simulink model "model"  (R2023b)
settings: Solver=ode23s  StartTime=0.0  StopTime=Tsim  MaxStep=1  RelTol=1e-3
values from neighbouring files (symbols this model uses):
  battery_capacity = 58    [parameters.m]    (also in vehicle_parameters.mat)
  CoG_height = 0.55    [parameters.m]    (also in vehicle_parameters.mat)
  Cx = 0.27    [parameters.m]    (also in vehicle_parameters.mat)
  e_motor_inverter_efficiency = 0.90    (= 0.9)    [parameters.m]    (also in vehicle_parameters.mat)
  f0 = 0.009    [parameters.m]    (also in vehicle_parameters.mat)
  f2 = 6.5 * 10^-6    (= 6.5e-06)    [parameters.m]    (also in vehicle_parameters.mat)
  F_mass_ratio = 0.5    [vehicle_parameters.mat]
  g = 9.81    [script.m]
  gear_ratio = 10.5    [parameters.m]    (also in vehicle_parameters.mat)
  inclination = 0    [script.m]
  J_to_Wh = 0.000277778    [script.m]    (also in vehicle_parameters.mat)
  kerb_weight = 1812    [parameters.m]    (also in vehicle_parameters.mat)
  max_speed = 16000    [parameters.m]    (also in vehicle_parameters.mat)
  max_torque = 310    [parameters.m]    (also in vehicle_parameters.mat)
  peak_power = 150*10^3    (= 150000)    [parameters.m]    (also in vehicle_parameters.mat)
  R_mass_ratio = 0.5    [vehicle_parameters.mat]
  rho = 1.204    [script.m]
  S = 2.36    [parameters.m]    (also in vehicle_parameters.mat)
  target = 300    [script.m]
  transmission_efficiency = 0.95    [parameters.m]    (also in vehicle_parameters.mat)
  velstart = 0    [script.m]
  wheel_radius = 0.359    [script.m]
  wheelbase = 2.77    [parameters.m]    (also in vehicle_parameters.mat)
settings Model: Creator=Matteo  LastModifiedBy=Matteo
settings DataIOCC: ReturnWorkspaceOutputs=off
settings DebuggingCC: SignalInfNanChecking=error

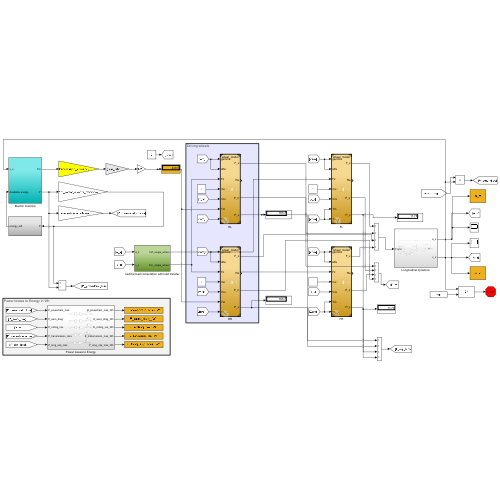
[thumbnail: Simulink's stored preview of the top-level diagram]
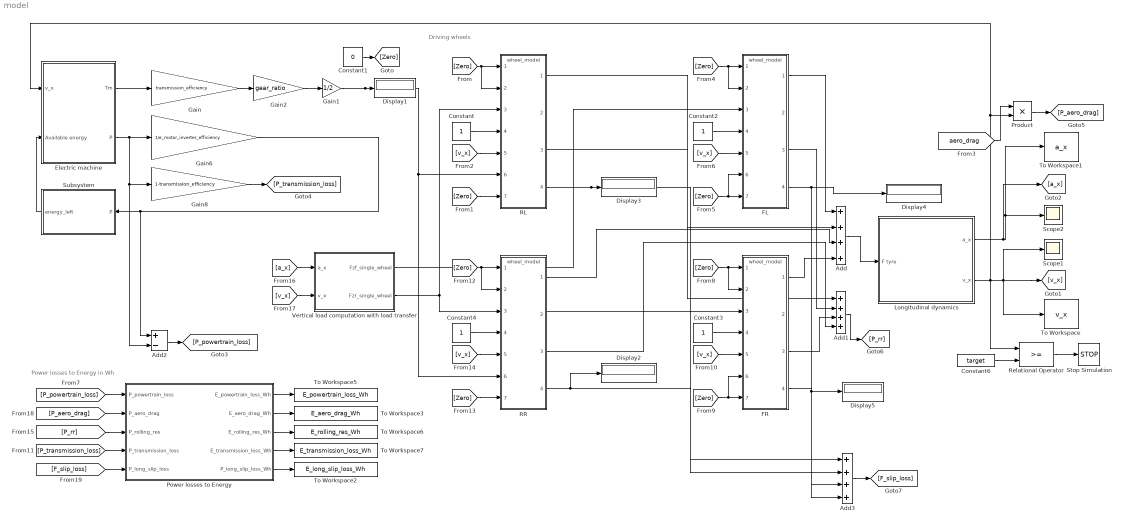
== system model ==
  note: Driving wheels
  note: Power losses to Energy in Wh
  Add : Sum  Inputs=++++
  Add1 : Sum  Inputs=++++
  Add2 : Sum  Inputs=+-
  Add3 : Sum  Inputs=++++
  Constant{,2..4} (4 alike) : Constant
  Constant1 : Constant  Value=0
  Constant6 : Constant  Value=target
  Display{1..5} (5 alike) : Display
  Electric machine : Subsystem
  FL : ModelReference  ModelNameDialog=wheel_model.slx  SimulationMode=Normal  ModelReferenceVersion=1.55
  FR : ModelReference  ModelNameDialog=wheel_model.slx  SimulationMode=Normal  ModelReferenceVersion=1.55
  Gain : Gain  Gain=transmission_efficiency
  Gain1 : Gain  Gain=1/2
  Gain2 : Gain  Gain=gear_ratio
  Gain6 : Gain  Gain=1/e_motor_inverter_efficiency
  Gain8 : Gain  Gain=1-transmission_efficiency
  Longitudinal dynamics : Subsystem
  Power losses to Energy : Subsystem
  Product : Product
  RL : ModelReference  ModelNameDialog=wheel_model.slx  SimulationMode=Normal  ModelReferenceVersion=1.55
  RR : ModelReference  ModelNameDialog=wheel_model.slx  SimulationMode=Normal  ModelReferenceVersion=1.55
  Relational Operator : RelationalOperator  OutDataTypeStr=boolean  RndMeth=Simplest  InputSameDT=off
  Scope1 : Scope
  Scope2 : Scope
  Stop Simulation : Stop
  Subsystem : Subsystem
  To Workspace : ToWorkspace  VariableName=v_x  SampleTime=-1
  To Workspace1 : ToWorkspace  VariableName=a_x  SampleTime=-1
  To Workspace2 : ToWorkspace  VariableName=E_long_slip_loss_Wh  SampleTime=-1
  To Workspace3 : ToWorkspace  VariableName=E_aero_drag_Wh  SampleTime=-1
  To Workspace5 : ToWorkspace  VariableName=E_powertrain_loss_Wh  SampleTime=-1
  To Workspace6 : ToWorkspace  VariableName=E_rolling_res_Wh  SampleTime=-1
  To Workspace7 : ToWorkspace  VariableName=E_transmission_loss_Wh  SampleTime=-1
  Vertical load computation with load transfer : Subsystem
  wires:
  [Zero] -> RL/2, RL/1
  Constant1/1 -> [Zero]
  Gain1/1 -> RL/6, RR/6, Display1/1
  Gain/1 -> Gain2/1
  Gain2/1 -> Gain1/1
  [Zero] -> RL/7
  [v_x] -> RL/5
  Constant/1 -> RL/4
  [Zero] -> FL/6, FL/7
  [Zero] -> FL/2, FL/1
  [v_x] -> FL/5
  Constant2/1 -> FL/4
  [v_x] -> FR/5
  [Zero] -> FR/2, FR/1
  Constant3/1 -> FR/4
  [Zero] -> FR/6, FR/7
  [v_x] -> RR/5
  [Zero] -> RR/2, RR/1
  Constant4/1 -> RR/4
  [Zero] -> RR/7
  Add/1 -> Longitudinal dynamics/1(F tyre)
  FL/1 -> Add/1
  FR/1 -> Add/4
  RR/1 -> Add/3
  RL/1 -> Add/2
  [a_x] -> Vertical load computation with load transfer/1(a_x)
  [v_x] -> Vertical load computation with load transfer/2(v_x)
  Vertical load computation with load transfer/1(Fzf_single_wheel) -> FR/3, FL/3
  Vertical load computation with load transfer/2(Fzr_single_wheel) -> RL/3, RR/3
  Longitudinal dynamics/1(a_x) -> To Workspace1/1, Scope2/1, [a_x]
  Relational Operator/1 -> Stop Simulation/1
  Longitudinal dynamics/2(v_x) -> Electric machine/1(v_x), Product/2, Relational Operator/1, Scope1/1, [v_x], To Workspace/1
  Constant6/1 -> Relational Operator/2
  Electric machine/1(Tm) -> Gain/1
  RR/3 -> Add1/4
  RL/3 -> Add1/1
  FL/3 -> Add1/2
  FR/3 -> Add1/3
  Add1/1 -> [P_rr]
  Subsystem/1(energy_left) -> Electric machine/2(Available energy)
  [aero_drag] -> Product/1
  RL/4 -> Display3/1, Add3/1
  RR/4 -> Display2/1, Add3/2
  FL/4 -> Display4/1, Add3/3
  FR/4 -> Display5/1, Add3/4
  Gain8/1 -> [P_transmission_loss]
  Product/1 -> [P_aero_drag]
  Electric machine/2(P) -> Add2/2, Gain8/1, Gain6/1
  Gain6/1 -> Subsystem/1(P), Add2/1
  Add2/1 -> [P_powertrain_loss]
  Add3/1 -> [F_slip_loss]
  [P_transmission_loss] -> Power losses to Energy/4(P_transmission_loss)
  Power losses to Energy/1(E_powertrain_loss_Wh) -> To Workspace5/1
  Power losses to Energy/5(P_long_slip_loss_Wh) -> To Workspace2/1
  Power losses to Energy/2(E_aero_drag_Wh) -> To Workspace3/1
  [F_slip_loss] -> Power losses to Energy/5(P_long_slip_loss)
  [P_aero_drag] -> Power losses to Energy/2(P_aero_drag)
  Power losses to Energy/4(E_transmission_loss_Wh) -> To Workspace7/1
  Power losses to Energy/3(E_rolling_res_Wh) -> To Workspace6/1
  [P_powertrain_loss] -> Power losses to Energy/1(P_powertrain_loss)
  [P_rr] -> Power losses to Energy/3(P_rolling_res)

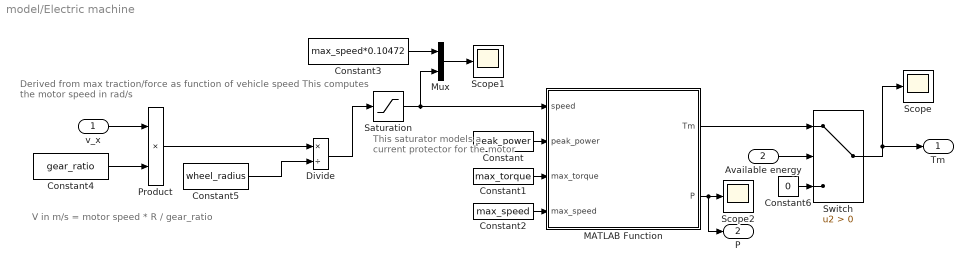
== system model/Electric machine ==
  note: This saturator models a current protector for the motor
  note: V in m/s = motor speed * R / gear_ratio
  note: Derived from max traction/force as function of vehicle speed
      | This computes the motor speed in rad/s
  v_x : Inport
  Available energy : Inport  Port=2
  Constant : Constant  Value=peak_power
  Constant1 : Constant  Value=max_torque
  Constant2 : Constant  Value=max_speed
  Constant3 : Constant  Value=max_speed*0.10472
  Constant4 : Constant  Value=gear_ratio
  Constant5 : Constant  Value=wheel_radius
  Constant6 : Constant  Value=0
  Divide : Product  Inputs=*/
  MATLAB Function : MATLAB Function  TreatAsAtomicUnit=on
  Mux : Mux  Inputs=2
  Product : Product
  Saturation : Saturate  UpperLimit=max_speed*0.10472*1  LowerLimit=-max_speed*0.10472*1
  Scope : Scope
  Scope1 : Scope
  Scope2 : Scope
  Switch : Switch  Criteria=u2 > Threshold  SaturateOnIntegerOverflow=off  InputSameDT=off
  Tm : Outport
  P : Outport  Port=2
  wires:
  Constant/1 -> MATLAB Function/2(peak_power)
  Constant1/1 -> MATLAB Function/3(max_torque)
  Constant2/1 -> MATLAB Function/4(max_speed)
  MATLAB Function/2(P) -> P/1, Scope2/1
  v_x/1 -> Product/1
  Constant4/1 -> Product/2
  Product/1 -> Divide/1
  Constant5/1 -> Divide/2
  Divide/1 -> Saturation/1
  Mux/1 -> Scope1/1
  Constant3/1 -> Mux/1
  Available energy/1 -> Switch/2
  Constant6/1 -> Switch/3
  Switch/1 -> Scope/1, Tm/1
  MATLAB Function/1(Tm) -> Switch/1
  Saturation/1 -> MATLAB Function/1(speed), Mux/2

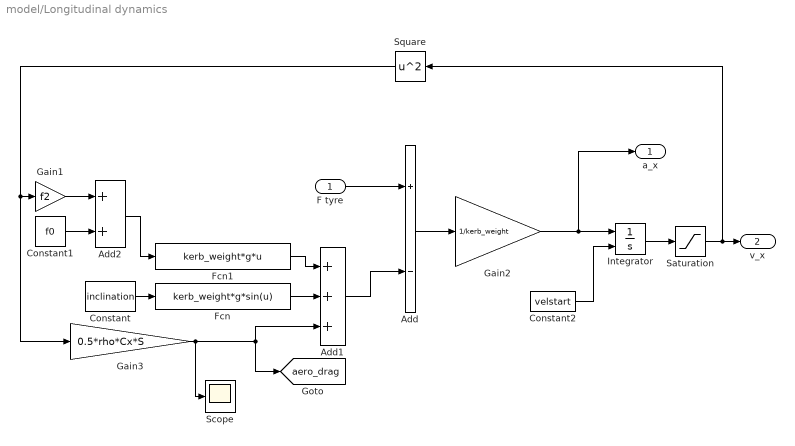
== system model/Longitudinal dynamics ==
  F tyre : Inport
  Add : Sum  Inputs=+-
  Add1 : Sum  Inputs=+++
  Add2 : Sum
  Constant : Constant  Value=inclination
  Constant1 : Constant  Value=f0
  Constant2 : Constant  Value=velstart
  Fcn : Fcn  Expr=kerb_weight*g*sin(u)
  Fcn1 : Fcn  Expr=kerb_weight*g*u
  Gain1 : Gain  Gain=f2
  Gain2 : Gain  Gain=1/kerb_weight
  Gain3 : Gain  Gain=0.5*rho*Cx*S
  Integrator : Integrator  InitialConditionSource=external  UpperSaturationLimit=500  LowerSaturationLimit=-500
  Saturation : Saturate  UpperLimit=inf  LowerLimit=0
  Scope : Scope
  Square : Math  Operator=square
  a_x : Outport
  v_x : Outport  Port=2
  tag scope: aero_drag=global
  wires:
  F tyre/1 -> Add/1
  Add1/1 -> Add/2
  Constant/1 -> Fcn/1
  Fcn/1 -> Add1/2
  Constant1/1 -> Add2/2
  Add/1 -> Gain2/1
  Gain2/1 -> Integrator/1, a_x/1
  Constant2/1 -> Integrator/2
  Square/1 -> Gain3/1, Gain1/1
  Gain1/1 -> Add2/1
  Add2/1 -> Fcn1/1
  Fcn1/1 -> Add1/1
  Gain3/1 -> Scope/1, [aero_drag], Add1/3
  Integrator/1 -> Saturation/1
  Saturation/1 -> Square/1, v_x/1

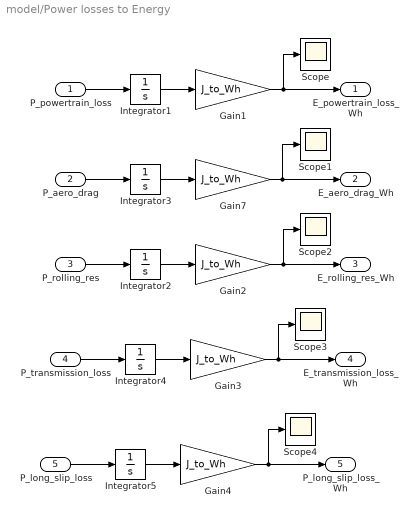
== system model/Power losses to Energy ==
  P_powertrain_loss : Inport
  P_aero_drag : Inport  Port=2
  P_rolling_res : Inport  Port=3
  P_transmission_loss : Inport  Port=4
  P_long_slip_loss : Inport  Port=5
  Gain{1..4,7} (5 alike) : Gain  Gain=J_to_Wh
  Integrator{1..5} (5 alike) : Integrator
  Scope{,1..4} (5 alike) : Scope
  E_powertrain_loss_Wh : Outport
  E_aero_drag_Wh : Outport  Port=2
  E_rolling_res_Wh : Outport  Port=3
  E_transmission_loss_Wh : Outport  Port=4
  P_long_slip_loss_Wh : Outport  Port=5
  wires:
  P_powertrain_loss/1 -> Integrator1/1
  Integrator3/1 -> Gain7/1
  P_aero_drag/1 -> Integrator3/1
  Integrator1/1 -> Gain1/1
  Gain1/1 -> Scope/1, E_powertrain_loss_Wh/1
  Gain7/1 -> Scope1/1, E_aero_drag_Wh/1
  Integrator2/1 -> Gain2/1
  P_rolling_res/1 -> Integrator2/1
  Gain2/1 -> Scope2/1, E_rolling_res_Wh/1
  Integrator4/1 -> Gain3/1
  P_transmission_loss/1 -> Integrator4/1
  Gain3/1 -> Scope3/1, E_transmission_loss_Wh/1
  Gain4/1 -> Scope4/1, P_long_slip_loss_Wh/1
  P_long_slip_loss/1 -> Integrator5/1
  Integrator5/1 -> Gain4/1

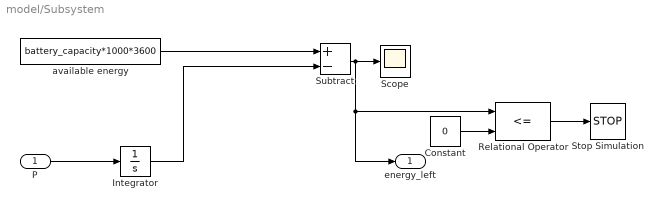
== system model/Subsystem ==
  P : Inport
  Constant : Constant  Value=0
  Integrator : Integrator
  Relational Operator : RelationalOperator  Operator=<=  OutDataTypeStr=boolean  RndMeth=Simplest  InputSameDT=off
  Scope : Scope
  Stop Simulation : Stop
  Subtract : Sum  Inputs=+-
  available energy : Constant  Value=battery_capacity*1000*3600
  energy_left : Outport
  wires:
  P/1 -> Integrator/1
  Integrator/1 -> Subtract/2
  available energy/1 -> Subtract/1
  Constant/1 -> Relational Operator/2
  Relational Operator/1 -> Stop Simulation/1
  Subtract/1 -> Relational Operator/1, energy_left/1, Scope/1

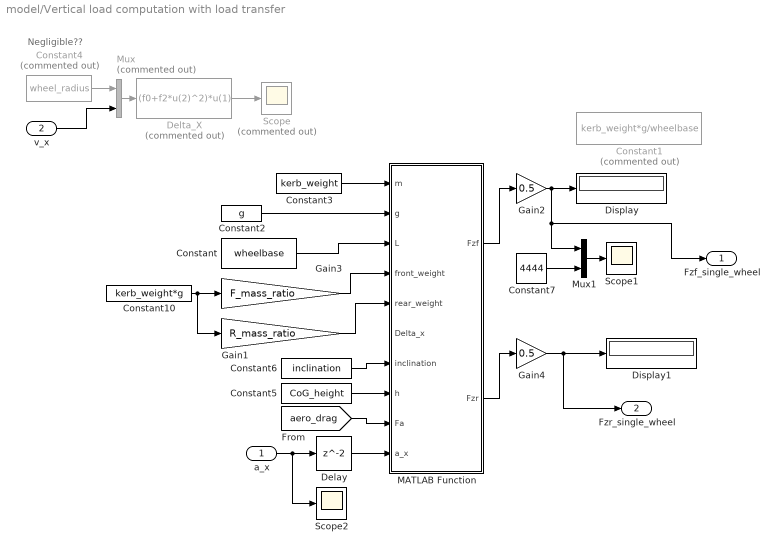
== system model/Vertical load computation with load transfer ==
  note: Negligible??
  a_x : Inport
  v_x : Inport  Port=2
  Constant : Constant  Value=wheelbase
  Constant1 : Constant  Commented=on  Value=kerb_weight*g/wheelbase
  Constant10 : Constant  Value=kerb_weight*g
  Constant2 : Constant  Value=g
  Constant3 : Constant  Value=kerb_weight
  Constant4 : Constant  Commented=on  Value=wheel_radius
  Constant5 : Constant  Value=CoG_height
  Constant6 : Constant  Value=inclination
  Constant7 : Constant  Value=4444
  Delay : Delay
  Delta_X : Fcn  Commented=on  Expr=(f0+f2*u(2)^2)*u(1)
  Display : Display
  Display1 : Display
  Gain1 : Gain  Gain=R_mass_ratio
  Gain2 : Gain  Gain=0.5
  Gain3 : Gain  Gain=F_mass_ratio
  Gain4 : Gain  Gain=0.5
  MATLAB Function : MATLAB Function  TreatAsAtomicUnit=on
  Mux : Mux  Commented=on  Inputs=2
  Mux1 : Mux  Inputs=2
  Scope : Scope  Commented=on
  Scope1 : Scope
  Scope2 : Scope
  Fzf_single_wheel : Outport
  Fzr_single_wheel : Outport  Port=2
  wires:
  Constant10/1 -> Gain1/1, Gain3/1
  Gain3/1 -> MATLAB Function/4(front_weight)
  Gain1/1 -> MATLAB Function/5(rear_weight)
  Constant/1 -> MATLAB Function/3(L)
  Constant2/1 -> MATLAB Function/2(g)
  Constant3/1 -> MATLAB Function/1(m)
  MATLAB Function/1(Fzf) -> Gain2/1
  MATLAB Function/2(Fzr) -> Gain4/1
  Mux/1 -> Delta_X/1
  Constant4/1 -> Mux/1
  v_x/1 -> Mux/2
  Delta_X/1 -> Scope/1
  Constant5/1 -> MATLAB Function/8(h)
  Constant6/1 -> MATLAB Function/7(inclination)
  [aero_drag] -> MATLAB Function/9(Fa)
  a_x/1 -> Scope2/1, Delay/1
  Gain4/1 -> Fzr_single_wheel/1, Display1/1
  Gain2/1 -> Fzf_single_wheel/1, Mux1/1, Display/1
  Delay/1 -> MATLAB Function/10(a_x)
  Constant7/1 -> Mux1/2
  Mux1/1 -> Scope1/1

== matlab function model/Electric machine/MATLAB Function ==
  data: speed input; Tm output; peak_power input; max_torque input; max_speed input; P output
function [Tm,P] = fcn(speed,peak_power,max_torque,max_speed)

transition_speed = peak_power/max_torque; % rad/s
max_speed_rad_s = max_speed*0.10472;


if speed <= transition_speed
   Tm = max_torque;
elseif speed > transition_speed && speed <= max_speed_rad_s
   Tm = peak_power/speed;
else
   Tm = 0;
end

P = Tm*speed;

end

== matlab function model/Vertical load computation with load transfer/MATLAB Function ==
  data: m input; Fzf output; g input; L input; Fzr output; front_weight input; rear_weight input; Delta_x input; inclination input; h input; Fa input; a_x input
function [Fzf,Fzr] = semi_wheel_bases(m,g,L, front_weight, rear_weight, Delta_x, inclination, h, Fa, a_x)

b = (front_weight*L)/(m*g);
a = (rear_weight*L)/(m*g);


Fzf = m*g/L * ( (b-Delta_x)*cos(inclination) - h*sin(inclination) - (Fa*h)/(m*g) - (a_x*h)/g );
Fzr = m*g/L * ( (a-Delta_x)*cos(inclination) - h*sin(inclination) - (Fa*h)/(m*g) - (a_x*h)/g );
